simulink model "rtwdemo_hyperlinks"  (Simulink 6.0)
settings: Solver=FixedStepDiscrete  StartTime=0.0  StopTime=48  FixedStep=1  RelTol=1e-3
libraries: rtwdemowidgets x2
settings Model: CovMetricSettings=d  Creator=The MathWorks Inc.  LastModifiedBy=batserve  ParamWorkspaceSource=ReferencedWorkspace  ExtModeTrigMode=oneshot  ExtModeArmWhenConnect=off  ExtModeAutoUpdateStatusClock=off
settings DataIOCC: LimitDataPoints=off  SaveFormat=StructureWithTime  SaveOutput=off  SaveTime=off  SignalLoggingName=sigsOut
settings OptimizationCC: InlineParams=on  EnforceIntegerDowncast=off  StateBitsets=on  DataBitsets=on  UseTempVars=on  ZeroExternalMemoryAtStartup=off  ZeroInternalMemoryAtStartup=off  InitFltsAndDblsToZero=off  NoFixptDivByZeroProtection=on  OptimizeModelRefInitCode=on  LifeSpan=1
settings DebuggingCC: CheckExecutionContextPreStartOutputMsg=on  CheckExecutionContextRuntimeOutputMsg=on  SolverPrmCheckMsg=none  IntegerOverflowMsg=none
settings ModelReferenceCC: UpdateModelReferenceTargets=IfOutOfDate
settings RTWCC: SystemTargetFile=ert.tlc  TLCOptions=-p0 -aWarnNonSaturatedBlocks=0  TemplateMakefile=ert_default_tmf  GenerateReport=on  RTWVerbose=off  ProcessScript=ert_make_rtw_hook  IncludeHyperlinkInReport=on  LaunchReport=on
settings CodeAppCC: ForceParamTrailComments=on  IgnoreCustomStorageClasses=off  SimulinkDataObjDesc=on  PrefixModelToSubsysFcnNames=off  CustomSymbolStr=$N$M  InsertBlockDesc=on
settings ERTTargetCC: TargetFcnLib=ansi_tfl_tmw.mat  GenFloatMathFcnCalls=ANSI_C  GenerateSampleERTMain=on  IncludeMdlTerminateFcn=off  SupportNonFinite=off  SupportComplex=off  InlinedParameterPlacement=NonHierarchical  RootIOFormat=Individual Arguments  ERTCustomFileTemplate=example_file_process.tlc  InitialValueSource=Model

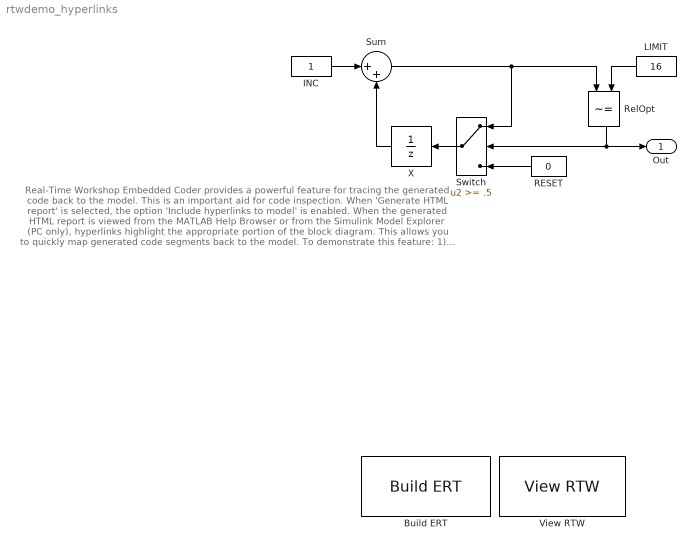
== system rtwdemo_hyperlinks ==
  note: Real-Time Workshop Embedded Coder provides a powerful feature for tracing the generated code
      | back to the model.  This is an important aid for code inspection.  When 'Generate HTML report'
      | is selected, the option 'Include hyperlinks to model' is enabled.  When the generated HTML
      | report is viewed from the MATLAB Help Browser or from the Simulink Model Explorer (PC only),
      | hyperlinks highlight the appropriate portion of the block diagram.  This allows you to quickly
      | map generated code segments back to the model.  To demonstrate this feature:
      |
      | 1) Open the Real-Time Workshop page by double-clicking the yellow button below
      | 2) Verify 'Generate HTML Report,' 'Include hyperlinks to model,' and 'Launch report
      |     report after code generation completes' options are selected
      | 3) Generate code by pressing the Build button, or double-click the blue button below
      | 4) Once the report is created, select the link for file rtwdemo_hyperlinks.c
      | 5) Select various hyperlinks in the code.  For example, /* Sum: '<Root>/Sum' */ is
      |     hyperlinked and sources back to the Sum block above.
  Build ERT : rtwdemowidgets/Build ERT  attrib_overrides={}
  INC : Constant  OutDataTypeMode=uint8
  LIMIT : Constant  Orientation=left  Value=16  OutDataTypeMode=uint8
  RESET : Constant  Orientation=left  Value=0  OutDataTypeMode=uint8
  RelOpt : RelationalOperator  Orientation=down  Operator=~=  InputSameDT=on
  Sum : Sum  Inputs=|++  InputSameDT=on
  Switch : Switch  Orientation=left  Threshold=.5  SaturateOnIntegerOverflow=on  InputSameDT=on
  View RTW : rtwdemowidgets/View RTW
  X : UnitDelay  Orientation=left  StateIdentifier=X
  Out : Outport
  wires:
  INC/1 -> Sum/1
  X/1 -> Sum/2
  Switch/1 -> X/1
  Sum/1 -> Switch/1, RelOpt/1
  LIMIT/1 -> RelOpt/2
  RESET/1 -> Switch/3
  RelOpt/1 -> Switch/2, Out/1
